simulink model "flightControlSystem"  (R2023b)
settings: Solver=ode3  StartTime=0  StopTime=TFinal  FixedStep=Ts  RelTol=1e-3  EnableMultiTasking=on
undefined symbols (not defined in the file): codertarget, Controller, DiscIntNeverNeededParam, Discrete, Estimator, g, gray, init, Sensors, Time, Ts, var_acc_angle_N, var_bias_gyr_N, var_gyro_p_N, Vehicle
libraries: simulink x38, slpidlib x4, ctrlSharedLib x4, sharedtransform x3, parrotlib x1
(part 3 of 3)

== matlab function flightControlSystem/Control System/Path Planning/calculate slope ==
  data: arr input; slopeOfLine output; zPos input; move output; right input; backtrackAmt input
function [slopeOfLine, move] = fcn(arr, zPos, right, backtrackAmt)
    persistent movementFreeTrial
    persistent lastSlope;
    persistent prevSlope;
    if (zPos < -1.095)
        if isempty(prevSlope)
            prevSlope = 1;
        end
        move = true;
        o = calculateSlope(arr, prevSlope, true, 10, 20);
        slopeOfLine = o(1);
        defined = o(2);
        if isempty(movementFreeTrial)
            movementFreeTrial = -1;
        end
        if isempty(lastSlope)
            lastSlope = -1;
        end
        if defined
            movementFreeTrial = 40;
            lastSlope = slopeOfLine;
        else
            
            if movementFreeTrial > 0
                disp("no line found!");
                slopeOfLine = lastSlope;
                movementFreeTrial = movementFreeTrial-1;
            else
                disp("recalculate slope!");
                %the drone will intially make the assumption that it is on
                %the red line. If this assumption causes issues later on I
                %will change this. The drone will search in the direction
                %of lastSlope for the first pixel to not be on the line(ie,
                %red) and it will move by half the line width backwards to
                %be at approximately the line's vertex. It will then get a
                %rough calculation of the slope which it can then use to
                %get the desiredN

                %this is an inefficent way to search for end of the line
                %but it's probably fine since it only happens rarely
                [numRow, numCol] = size(arr);
                midCol = numCol / 2;
                midRow = numRow / 2;
                lineWidth = 19;
                lineRadius = lineWidth / 2.0;
                x = 0;
                y = 0;
                for i=floor(lineRadius):1:midCol
                    if right
                        j = i;
                    else
                        j = -i;
                    end

                    x = midCol + j;
                    y = floor(numRow-(midRow+(prevSlope*j)));
                    if ~arr(y, x)
                        if right
                            j = j-backtrackAmt;
                        else
                            j = j+backtrackAmt;
                        end
                        x = midCol + j;
                        y = floor(numRow-(midRow+(prevSlope*j)));
                        break;
                    end
                end
                if ~arr(y, x)
                    disp("this shoudln't happen!!")
                end
                xOffset = x-midCol
                yOffset = y-midRow
                
                prevSlope = calculateNewSlope(arr, xOffset, yOffset, prevSlope, 1, 5);
                disp("prev");
                disp(prevSlope);
                movementFreeTrial = 40;
                error("stop")
                
                


            end
        end
    else
        move = false;
        slopeOfLine = -1;
    end
end

function newSlope = calculateNewSlope(arr, xOffset, yOffset, oldSlope, oldSlopeTolerance, pixelTolerance)
    xOffset = xOffset*2;
    yOffset = yOffset*2;
    lineWidth = 19;
    lineRadius = lineWidth/2;
    [numRow, numCol] = size(arr);
    arrWidth = numCol - abs(xOffset);
    arrHeight = numRow - abs(yOffset);
    perimeterPixels = ((arrHeight-2)*2)+(arrWidth*2);
    newSlope = 0;
    n=1;
    while (n <= perimeterPixels)
        currentPixel = searchPerimeter(n, numCol, numRow, xOffset, yOffset);
        x = currentPixel(1);
        y = currentPixel(2);
        if ~arr(y, x)
            n = n+1;
            continue
        end
        slope = getSlope((x-(arrWidth/2))/lineRadius, ((arrHeight/2)-y)/lineRadius);
        expectedPixels = pixelsIntersected(slope, lineWidth, arrWidth, arrHeight);
        pixCount = 0;
        
        while (arr(y, x))
            pixCount = pixCount+1;
            n = n+1;
            currentPixel = searchPerimeter(mod(n-1, perimeterPixels)+1, numCol, numRow, xOffset, yOffset);
            x = currentPixel(1);
            y = currentPixel(2);
        end
        % can't be bothered to use demorgan's law
        if  abs(slope-oldSlope) > oldSlopeTolerance && (pixCount > expectedPixels-pixelTolerance && pixCount < expectedPixels+pixelTolerance)
            newSlope = slope;
            disp(newSlope);
            disp(x)
            disp(y)
            disp(n)
        end
        n = n+1;
    end
    if newSlope == 0
        disp("this shouldn't happen");
    end
end

    
%vertSlope should be the slope calculated by the new line function
%right is a boolean which determines whether the slope should
%represent the right end of the slope or the left end
function [output] = calculateSlope(arr, vertSlope, right, pixelTolerance, nTolerance)
    persistent desiredN;

    [numRow, numCol] = size(arr);
    midCol = numCol / 2;
    midRow = numRow / 2;
    % lineWidth is likely 19
    lineWidth = 19;
    lineRadius = lineWidth / 2.0;
    rowCenter = numRow / 2.0;
    current = arr(1, 1);
    lineEnd = true;
    perimeterPixels = ((numRow-2)*2)+(numCol*2);
    slope = 0;
    defined = false;
    n=1;
    if isempty(desiredN)
        desiredN = floor(slopeToN(vertSlope, numCol, numRow, lineRadius, right));
    end

    %remake this with for loop
    for b = desiredN-nTolerance:1:desiredN+nTolerance
        n = mod(b-1, perimeterPixels)+1;
        currentPixel = searchPerimeter(n, numCol, numRow, 0, 0);
        x = currentPixel(1);
        y = currentPixel(2);

        possibleSlope = getSlope((x-(numCol/2))/lineRadius, ((numRow/2)-y)/lineRadius);
        disp(possibleSlope)
        expectedPixels = pixelsIntersected(possibleSlope, lineWidth, numCol, numRow);
        pixCount = 0;
        while (arr(currentPixel(2), currentPixel(1)))
            pixCount = pixCount+1;
            n = n+1;
            currentPixel = searchPerimeter(mod(n-1, perimeterPixels)+1, numCol, numRow, 0, 0);
        end
        
        if (pixCount > expectedPixels-pixelTolerance && pixCount < expectedPixels+pixelTolerance)
            slope = possibleSlope;
            defined = true;
            break;
        end
    end
    output = [slope, defined];

end
function desiredN = slopeToN(slope, numCol, numRow, lineRadius, right)
    midCol = numCol / 2;
    midRow = numRow / 2;
    %basically here I need to figure out if the line is the one
    %from the slope by seeing how many pixels off the current line
    %is from the original one. The pixels of the current line is
    %given already(in n) and in pixCount, however the pixels of the
    %original line need to be recalculated(this needs to be done
    %anyway to deal with array size changes). The computer doesn't
    %need the start and end of both of them, it can just compare
    %the difference in index of the right edges for both lines. To
    %get the right edge index of the calculated slope is, however,
    %much easier said then done: first, the position where the
    %right edge intersects with the edge of the camera needs to be
    %calculated. This can be done by finding the y intercept by
    %doing some math(see this desmos graph:
    %https://www.desmos.com/calculator/vv2ejgyblp) and then
    %determine whether or not said slope will intercept a
    %left/right edge or a top/bottom edge by looking at whether
    %it's greater than the height of the screen divided by its
    %width. If you then do plug in numbers accordingly you should
    %get the position of the right edge. In the same if/else
    %statement for determining top/right, calculate index by
    %reverse engineering the search perimeter function, it should
    %be easier.
    
    %if top or bottom
    
    yInt = -(lineRadius*sqrt(slope^2+1));
    if (abs(slope) > 0.9106)
        %checks for top or bottom
    
        if ((slope > 0) == right)
            %this is for top, therefore the y's index is 1 and its
            %y position(used for calculating slope) should be half
            %the height this can be pluged into the desmos equation
            %to get the x position which can then be translated to
            %slope
            xPos = (midRow-yInt)/slope;
            %since it's on the top I can translate x position to
            %index simply by flipping it, note that the index
            %starts at 1 so I'll need to add one.
            desiredN = numCol-(xPos+midCol)+1;
    
        else
            %this is for bottom
            xPos = ((midRow*-1)-yInt)/slope;
            desiredN = numCol+(numRow-1)+(xPos+midCol);
    
        end
    
    
        %if left or right
    else
        if (right)
            yPos = (slope*midCol)+yInt;
            desiredN = (numCol*2)+(numRow-2)+(yPos+midRow)-1;
        else
            yPos = (slope*midCol*-1)+yInt;
            desiredN = numCol+(numRow-(yPos+midRow))+1;
        end
    end
end

function slope = getSlope(x, y)
    % this is a gross overcomplication on multiple levels as per usual
    slope = 0;
    if (x^2 + y^2) >= 1
        d = sqrt(x^2 + y^2 - 1);
        slope = ((y*d+x)/(x*d-y));
    end
end
function output = searchPerimeter(n, numCol, numRow, xOffset, yOffset)
    arrWidth = numCol - abs(xOffset);
    arrHeight = numRow - abs(yOffset);
    x = 0;
    y = 0;
    %this is for the bottom and top of the rectangle, when this is true, x
    %is changing and y is fixed
    %n starts at 1
    if mod(n-1, arrWidth+arrHeight-2) < arrWidth
        %this is bottom of rectangle
        if n > arrWidth
            y = arrHeight;
            x = n-(arrHeight+arrWidth)+2;
        else
            %this is for the top
            y = 1;
            x = arrWidth-n+1;
        end
    else
        %this is for when its not the bottom or top of rectangle, so one of
        %the sides, notice the top and bottom get priority for corner
        %pixelsstoredRegion

        %this is for the left side
        if n <= (arrHeight+arrWidth)
            x = 1;
            y = n-arrWidth+2;
        else
            %right side
            x = arrWidth;
            y = (((arrWidth*2)+(arrHeight-2)*2)-n)+2;
        end
    end

    x = x+max(0, xOffset);
    y = y+max(0, yOffset);
    output = [x, y];
end

function pixels = pixelsIntersected(m, w, arrWidth, arrHeight)
    changeSlope = arrHeight/arrWidth;
    %this doesn't quite calculate the right value for the corners since it
    %should be calculating the height and width of the line's intersecion
    %with the surrounding rectangle for the cases in which the line
    %intersects the corners, however, I'm lazy and hoping that this is a
    %good enough approximation since the height and width of the rectangle
    %are typically somewhat close.
    if abs(m) > changeSlope
        pixels = abs((w*sqrt(m^2+1))/m);
    else
        pixels = w*(sqrt(m^2+1));
    end
end

== matlab function flightControlSystem/Image Processing System/MATLAB Function1 ==
  data: red output; arr input; xOffset input; yOffset input; nextN output; n input
function [red, nextN] = fcn(arr, xOffset, yOffset, n)
    xOffset = xOffset*2;
    yOffset = yOffset*2;
    lineWidth = 19;
    [numRow, numCol] = size(arr);
    arrWidth = numCol - abs(xOffset);
    arrHeight = numRow - abs(yOffset);
    n = 1;
    x = 0;
    y = 0;
    %n = floor(slopeToN(2, numCol, numRow, lineWidth/2.0, true));

    %this is for the bottom and top of the rectangle, when this is true, x
    %is changing and y is fixed
    %n starts at 1
    if mod(n-1, arrWidth+arrHeight-2) < arrWidth
        %this is bottom of rectangle
        if n > arrWidth
            y = arrHeight;
            x = n-(arrHeight+arrWidth)+2;
        else
            %this is for the top
            y = 1;
            x = arrWidth-n+1;
        end
    else
        %this is for when its not the bottom or top of rectangle, so one of
        %the sides, notice the top and bottom get priority for corner
        %pixels

        %this is for the left side
        if n <= (arrHeight+arrWidth)
            x = 1;
            y = n-arrWidth+2;
        else
            %right side
            x = arrWidth;
            y = (((arrWidth*2)+(arrHeight-2)*2)-n)+2;
        end
    end

    x = x+max(0, xOffset);
    y = y+max(0, yOffset);
    red = zeros(120, 160, 'uint8');
    red(y, x) = 255;
    red(floorDiv(arrHeight, 2)+max(0, yOffset),floorDiv(arrWidth, 2)+max(0, xOffset)) = 255;
    %slope = getSlope((x-(arrWidth/2))/(lineWidth/2), ((arrHeight/2)-y)/(lineWidth/2));
    %disp(slope);
    %estimatedXPixels = pixelsIntersected(slope, lineWidth, false);
    %disp(estimatedXPixels);
    nextN = n+1;
end

function desiredN = slopeToN(slope, numCol, numRow, lineRadius, right)
    midCol = numCol / 2;
    midRow = numRow / 2;
    %basically here I need to figure out if the line is the one
    %from the slope by seeing how many pixels off the current line
    %is from the original one. The pixels of the current line is
    %given already(in n) and in pixCount, however the pixels of the
    %original line need to be recalculated(this needs to be done
    %anyway to deal with array size changes). The computer doesn't
    %need the start and end of both of them, it can just compare
    %the difference in index of the right edges for both lines. To
    %get the right edge index of the calculated slope is, however,
    %much easier said then done: first, the position where the
    %right edge intersects with the edge of the camera needs to be
    %calculated. This can be done by finding the y intercept by
    %doing some math(see this desmos graph:
    %https://www.desmos.com/calculator/vv2ejgyblp) and then
    %determine whether or not said slope will intercept a
    %left/right edge or a top/bottom edge by looking at whether
    %it's greater than the height of the screen divided by its
    %width. If you then do plug in numbers accordingly you should
    %get the position of the right edge. In the same if/else
    %statement for determining top/right, calculate index by
    %reverse engineering the search perimeter function, it should
    %be easier.
    
    %if top or bottom
    
    yInt = -(lineRadius*sqrt(slope^2+1));
    if (abs(slope) > 0.9106)
        %checks for top or bottom
    
        if ((slope > 0) == right)
            %this is for top, therefore the y's index is 1 and its
            %y position(used for calculating slope) should be half
            %the height this can be pluged into the desmos equation
            %to get the x position which can then be translated to
            %slope
            xPos = (midRow-yInt)/slope;
            %since it's on the top I can translate x position to
            %index simply by flipping it, note that the index
            %starts at 1 so I'll need to add one.
            desiredN = numCol-(xPos+midCol)+1;
    
        else
            %this is for bottom
            xPos = ((midRow*-1)-yInt)/slope;
            desiredN = numCol+(numRow-1)+(xPos+midCol);
    
        end
    
    
        %if left or right
    else
        if (right)
            yPos = (slope*midCol)+yInt;
            desiredN = (numCol*2)+(numRow-2)+(yPos+midRow)-1;
        else
            yPos = (slope*midCol*-1)+yInt;
            desiredN = numCol+(numRow-(yPos+midRow))+1;
        end
    end
end

function slope = getSlope(x, y)
    % this is a gross overcomplication on multiple levels as per usual
    distSquared = x^2 + y^2;
    l = sqrt(distSquared - 1);
    slope = (y - ((y - x * l) / distSquared)) / (x - ((x + y * l) / distSquared));
end
function pixels = pixelsIntersected(m, w, arrWidth, arrHeight)
    changeSlope = arrHeight/arrWidth;
    %this doesn't quite calculate the right value for the corners since it
    %should be calculating the height and width of the line's intersecion
    %with the surrounding rectangle for the cases in which the line
    %intersects the corners, however, I'm lazy and hoping that this is a
    %good enough approximation since the height and width of the rectangle
    %are typically somewhat close.
    if abs(slope) > changeSlope
        pixels = abs((w*sqrt(m^2+1))/m);
    else
        pixels = w*(sqrt(m^2+1));
    end
end
